simulink model "example1"  (R2017b)
settings: Solver=ode45  StartTime=0.0  StopTime=10.0  RelTol=1e-3
settings Model: Creator=jeddelan  LastModifiedBy=JEDDELAN
settings DataIOCC: LimitDataPoints=on  SaveFormat=Array  SignalLoggingSaveFormat=ModelDataLogs
settings OptimizationCC: BlockReduction=off  BooleanDataType=off  LifeSpan=inf
settings DebuggingCC: SaveWithParameterizedLinksMsg=none  UnderspecifiedInitializationDetection=Classic  MergeDetectMultiDrivingBlocksExec=none  SignalResolutionControl=TryResolveAllWithWarning  MultiTaskDSMMsg=warning  MultiTaskCondExecSysMsg=none  StrictBusMsg=None  SFUnexpectedBacktrackingDiag=warning  SFNoUnconditionalDefaultTransitionDiag=warning  SFExecutionAtInitializationDiag=none
settings HardwareCC: ProdBitPerPointer=32  ProdBitPerSizeT=32  ProdBitPerPtrDiffT=32  ProdLargestAtomicFloat=None  ProdIntDivRoundTo=Undefined  ProdEndianess=Unspecified  ProdWordSize=32  ProdHWDeviceType=32-bit Generic  TargetUnknown=on
settings ModelReferenceCC: PropagateSignalLabelsOutOfModel=off
settings CodeAppCC: StateflowObjectComments=on
settings GRTTargetCC: TargetLangStandard=C89/C90 (ANSI)  GeneratePreprocessorConditionals=Disable all
settings ConfigComp: CovMetricSettings=dw  CovHtmlReporting=on  CovSaveCumulativeToWorkspaceVar=on  CovSaveSingleToWorkspaceVar=on  CovExternalEMLEnable=off

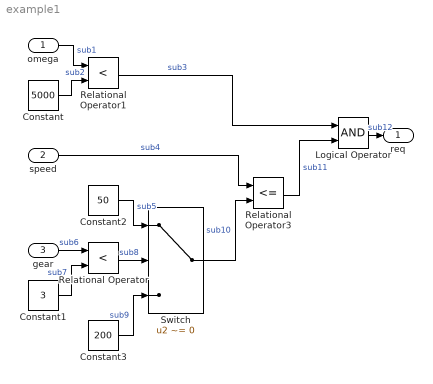
== system example1 ==
  omega : Inport
  speed : Inport  Port=2
  gear : Inport  Port=3
  Constant : Constant  Value=5000
  Constant1 : Constant  Value=3
  Constant2 : Constant  Value=50
  Constant3 : Constant  Value=200
  Logical Operator : Logic  AllPortsSameDT=off  OutDataTypeStr=boolean
  Relational Operator : RelationalOperator  Operator=<  OutDataTypeStr=boolean  RndMeth=Nearest
  Relational Operator1 : RelationalOperator  Operator=<  OutDataTypeStr=boolean  RndMeth=Nearest
  Relational Operator3 : RelationalOperator  Operator=<=  OutDataTypeStr=boolean  RndMeth=Nearest
  Switch : Switch  Criteria=u2 ~= 0
  req : Outport
  wires:
  gear/1 -> Relational Operator/1  "sub6"
  Constant1/1 -> Relational Operator/2  "sub7"
  Relational Operator/1 -> Switch/2  "sub8"
  omega/1 -> Relational Operator1/1  "sub1"
  Constant/1 -> Relational Operator1/2  "sub2"
  Constant3/1 -> Switch/3  "sub9"
  Constant2/1 -> Switch/1  "sub5"
  Switch/1 -> Relational Operator3/2  "sub10"
  Relational Operator1/1 -> Logical Operator/1  "sub3"
  Logical Operator/1 -> req/1  "sub12"
  speed/1 -> Relational Operator3/1  "sub4"
  Relational Operator3/1 -> Logical Operator/2  "sub11"
